simulink model "allocator_simulation"  (R2018b)
settings: Solver=VariableStepAuto  StartTime=0.0  StopTime=400  RelTol=1e-3
undefined symbols (not defined in the file or in its folder): fswParams
libraries: rigid_body_dynamics_lib x2, PD_Controller_Lib x1, null_allocation_lib x1, quat_kinematics_lib x1, reaction_wheel_assembly_lib x1, rwa_allocation_lib x1, two_norm x1
settings Model: Creator=Nick's PC  LastModifiedBy=Nick's PC

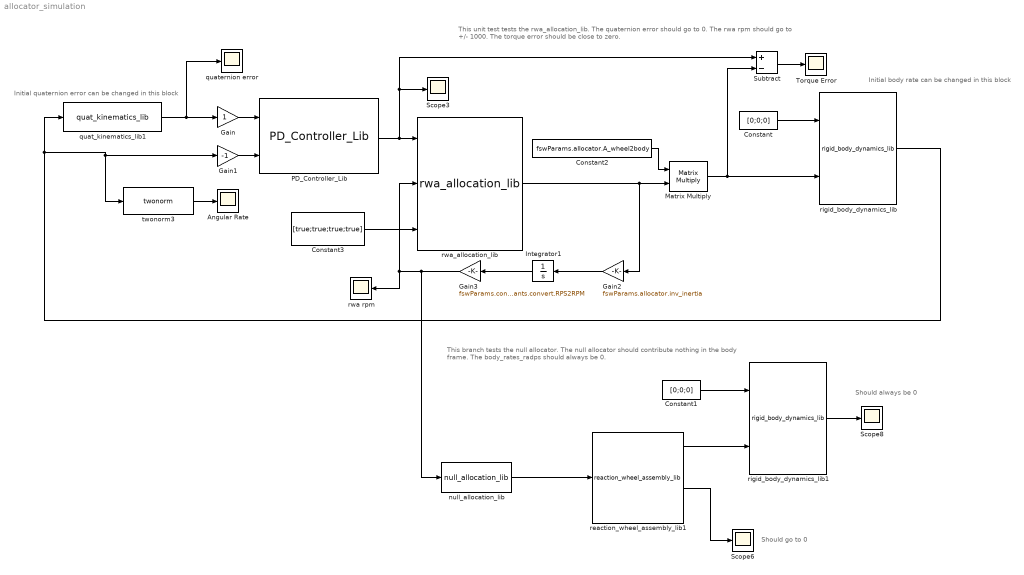
== system allocator_simulation ==
  note: Initial body rate can be changed in this block
  note: Initial quaternion error can be changed in this block
  note: Should go to 0
  note: Should always be 0
  note: This branch tests the null allocator. The null allocator should contribute nothing in the body frame. The body_rates_radps should always be 0.
  note: This unit test tests the rwa_allocation_lib. The quaternion error should go to 0. The rwa rpm should go to +/- 1000. The torque error should be close to zero.
  Angular Rate : Scope
  Constant : Constant  Value=[0;0;0]
  Constant1 : Constant  Value=[0;0;0]
  Constant2 : Constant  Value=fswParams.allocator.A_wheel2body
  Constant3 : Constant  Value=[true;true;true;true]
  Gain : Gain
  Gain1 : Gain  Gain=-1
  Gain2 : Gain  Gain=fswParams.allocator.inv_inertia
  Gain3 : Gain  Gain=fswParams.constants.convert.RPS2RPM
  Integrator1 : Integrator
  Matrix Multiply : Product  Multiplication=Matrix(*)
  PD_Controller_Lib : PD_Controller_Lib/PD_Controller_Lib  SystemSampleTime=-1
  Scope3 : Scope
  Scope6 : Scope
  Scope8 : Scope
  Subtract : Sum  Inputs=+-
  Torque Error : Scope
  null_allocation_lib : null_allocation_lib/null_allocation_lib  SystemSampleTime=-1
  quat_kinematics_lib1 : quat_kinematics_lib/quat_kinematics_lib  SystemSampleTime=-1
  quaternion error : Scope
  reaction_wheel_assembly_lib1 : reaction_wheel_assembly_lib/reaction_wheel_assembly_lib  SystemSampleTime=-1
  rigid_body_dynamics_lib : rigid_body_dynamics_lib/rigid_body_dynamics_lib  SystemSampleTime=-1
      link override Integrator: InitialCondition=simParams.initialConditions.w_body_radps
      link override Integrator1: InitialCondition=simParams.initialConditions.rwa.h_body_Nms
  rigid_body_dynamics_lib1 : rigid_body_dynamics_lib/rigid_body_dynamics_lib  SystemSampleTime=-1
  rwa rpm : Scope
  rwa_allocation_lib : rwa_allocation_lib/rwa_allocation_lib  SystemSampleTime=-1
  twonorm3 : two_norm/twonorm  SystemSampleTime=-1
  wires:
  Constant/1 -> rigid_body_dynamics_lib/1
  rwa_allocation_lib/1 -> Gain2/1, Matrix Multiply/2
  quat_kinematics_lib1/1 -> Gain/1, quaternion error/1
  Gain/1 -> PD_Controller_Lib/1
  Gain1/1 -> PD_Controller_Lib/2
  rigid_body_dynamics_lib/1 -> Gain1/1, twonorm3/1, quat_kinematics_lib1/1
  null_allocation_lib/1 -> reaction_wheel_assembly_lib1/1
  reaction_wheel_assembly_lib1/1 -> rigid_body_dynamics_lib1/2
  Constant1/1 -> rigid_body_dynamics_lib1/1
  reaction_wheel_assembly_lib1/3 -> Scope6/1
  rigid_body_dynamics_lib1/1 -> Scope8/1
  twonorm3/1 -> Angular Rate/1
  PD_Controller_Lib/1 -> Subtract/1, Scope3/1, rwa_allocation_lib/1
  Subtract/1 -> Torque Error/1
  Constant2/1 -> Matrix Multiply/1
  Gain2/1 -> Integrator1/1
  Constant3/1 -> rwa_allocation_lib/3
  Integrator1/1 -> Gain3/1
  Matrix Multiply/1 -> rigid_body_dynamics_lib/2, Subtract/2
  Gain3/1 -> null_allocation_lib/1, rwa rpm/1, rwa_allocation_lib/2
